simulink model "NoC_4x4x3"  (R2015a)
settings: Solver=ode45  StartTime=0.0  StopTime=10.0  RelTol=1e-3
undefined symbols (not defined in the file or in its folder): des, SELECT
undefined symbols (not defined in the file): MAX, MIN, T
libraries: simulink x48
(part 1 of 12)
settings Model: Creator=Nejib  LastModifiedBy=Nejib

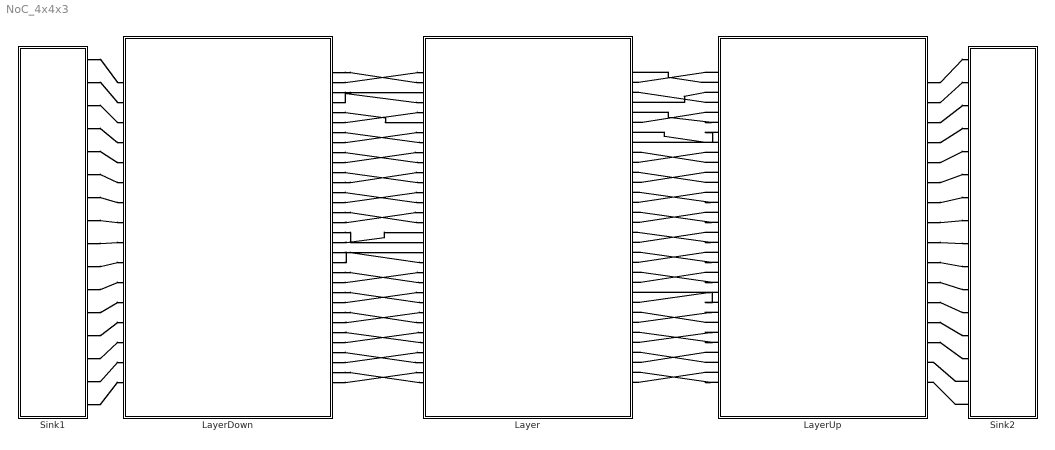
== system NoC_4x4x3 ==
  Layer : Subsystem
  LayerDown : Subsystem
  LayerUp : Subsystem
  Sink1 : Subsystem
      mask Display: fprintf('SINK')
  Sink2 : Subsystem
      mask Display: fprintf('SINK')
  connections:
  LayerUp/LConn1 -- Layer/RConn2
  LayerUp/LConn2 -- Layer/RConn1
  LayerUp/LConn3 -- Layer/RConn4
  LayerUp/LConn4 -- Layer/RConn3
  LayerUp/LConn5 -- Layer/RConn6
  LayerUp/LConn6 -- Layer/RConn5
  LayerUp/LConn7 -- Layer/RConn8
  LayerUp/LConn8 -- Layer/RConn7
  LayerUp/LConn9 -- Layer/RConn10
  LayerUp/LConn10 -- Layer/RConn9
  LayerUp/LConn11 -- Layer/RConn12
  LayerUp/LConn12 -- Layer/RConn11
  LayerUp/LConn13 -- Layer/RConn14
  LayerUp/LConn14 -- Layer/RConn13
  LayerUp/LConn16 -- Layer/RConn15
  LayerUp/LConn15 -- Layer/RConn16
  LayerUp/LConn17 -- Layer/RConn18
  LayerUp/LConn18 -- Layer/RConn17
  LayerUp/LConn19 -- Layer/RConn20
  LayerUp/LConn20 -- Layer/RConn19
  LayerUp/LConn21 -- Layer/RConn22
  LayerUp/LConn22 -- Layer/RConn21
  LayerUp/LConn24 -- Layer/RConn23
  LayerUp/LConn23 -- Layer/RConn24
  LayerUp/LConn25 -- Layer/RConn26
  LayerUp/LConn26 -- Layer/RConn25
  LayerUp/LConn27 -- Layer/RConn28
  LayerUp/LConn28 -- Layer/RConn27
  LayerUp/LConn29 -- Layer/RConn30
  LayerUp/LConn30 -- Layer/RConn29
  LayerUp/LConn31 -- Layer/RConn32
  LayerUp/LConn32 -- Layer/RConn31
  LayerDown/RConn27 -- Layer/LConn28
  LayerDown/RConn25 -- Layer/LConn26
  LayerDown/RConn18 -- Layer/LConn17
  LayerDown/RConn12 -- Layer/LConn11
  LayerDown/RConn21 -- Layer/LConn22
  LayerDown/RConn10 -- Layer/LConn9
  LayerDown/RConn14 -- Layer/LConn13
  LayerDown/RConn32 -- Layer/LConn31
  LayerDown/RConn5 -- Layer/LConn6
  LayerDown/RConn23 -- Layer/LConn24
  LayerDown/RConn19 -- Layer/LConn20
  LayerDown/RConn15 -- Layer/LConn16
  LayerDown/RConn6 -- Layer/LConn5
  LayerDown/RConn2 -- Layer/LConn1
  LayerDown/RConn1 -- Layer/LConn2
  LayerDown/RConn3 -- Layer/LConn4
  LayerDown/RConn4 -- Layer/LConn3
  LayerDown/RConn8 -- Layer/LConn7
  LayerDown/RConn7 -- Layer/LConn8
  LayerDown/RConn9 -- Layer/LConn10
  LayerDown/RConn11 -- Layer/LConn12
  LayerDown/RConn13 -- Layer/LConn14
  LayerDown/RConn16 -- Layer/LConn15
  LayerDown/RConn17 -- Layer/LConn18
  LayerDown/RConn20 -- Layer/LConn19
  LayerDown/RConn22 -- Layer/LConn21
  LayerDown/RConn24 -- Layer/LConn23
  LayerDown/RConn26 -- Layer/LConn25
  LayerDown/RConn28 -- Layer/LConn27
  LayerDown/RConn30 -- Layer/LConn29
  LayerDown/RConn29 -- Layer/LConn30
  LayerDown/RConn31 -- Layer/LConn32
  LayerUp/RConn2 -- Sink2/LConn1
  LayerUp/RConn4 -- Sink2/LConn2
  LayerUp/RConn6 -- Sink2/LConn3
  LayerUp/RConn8 -- Sink2/LConn4
  LayerUp/RConn10 -- Sink2/LConn5
  LayerUp/RConn12 -- Sink2/LConn6
  LayerUp/RConn14 -- Sink2/LConn7
  LayerUp/RConn16 -- Sink2/LConn8
  LayerUp/RConn18 -- Sink2/LConn9
  LayerUp/RConn20 -- Sink2/LConn10
  LayerUp/RConn22 -- Sink2/LConn11
  LayerUp/RConn24 -- Sink2/LConn12
  LayerUp/RConn26 -- Sink2/LConn13
  LayerUp/RConn28 -- Sink2/LConn14
  Sink2/LConn15 -- LayerUp/RConn30
  Sink2/LConn16 -- LayerUp/RConn32
  Sink1/LConn1 -- LayerDown/LConn2
  Sink1/LConn2 -- LayerDown/LConn4
  Sink1/LConn3 -- LayerDown/LConn6
  Sink1/LConn4 -- LayerDown/LConn8
  Sink1/LConn5 -- LayerDown/LConn10
  Sink1/LConn6 -- LayerDown/LConn12
  Sink1/LConn7 -- LayerDown/LConn14
  Sink1/LConn8 -- LayerDown/LConn16
  Sink1/LConn9 -- LayerDown/LConn18
  Sink1/LConn10 -- LayerDown/LConn20
  Sink1/LConn11 -- LayerDown/LConn22
  Sink1/LConn12 -- LayerDown/LConn24
  Sink1/LConn13 -- LayerDown/LConn26
  Sink1/LConn14 -- LayerDown/LConn28
  Sink1/LConn15 -- LayerDown/LConn30
  Sink1/LConn16 -- LayerDown/LConn32

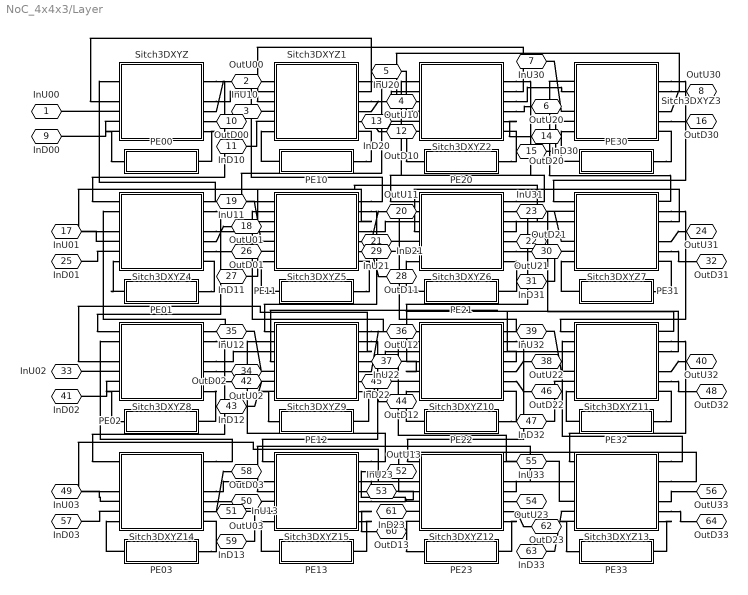
== system NoC_4x4x3/Layer ==
  PE00 : Subsystem  mask{ME=[1 1 2], D=5, SEED=100, tt=Uniform, MINU=MIN, MAXU=MAX, REGULAR=T, A=100, B=15, Router='Corner_Mean_Z2', Loss='Corner_Loss_Z2', N='Corner_N_Z2'}
      mask prompts: ME "Addresse"; D "Startup time"; tt "Traffic Type"; MINU "Min"; MAXU "Max"; REGULAR "T"; A "Lambda 1"; B "Lambda 2"; Router "Mean delay"; Loss "Instant number of lost flits"; N "Number of departed flits"
      mask init:
      | set_param([gcb '/Router'],'VariableName',Router)
      | set_param([gcb '/Loss'],'VariableName',Loss)
      | set_param([gcb '/N'],'VariableName',N)
      | V=1:4;
      | V_X = V(V~=ME(1));
      | V_Y = V(V~=ME(2));
      | V_Z = V(V~=ME(3));
      mask TypeOptions tt: Periodic | Uniform | MMPP
      mask Callback tt:
      | maskStr = get_param(gcb,'tt');
      | msk = Simulink.Mask.get(gcbh);
      | %p = msk.Parameters;
      | %
      | % P = msk.getParameter('MINU');
      | % U = msk.getParameter('MAXU');
      | % M = msk.getParameter('REGULAR');
      | 
      | P = msk.getDialogControl('Periodic');
      | U = msk.getDialogControl('Uniform');
      | M = msk.getDialogControl('MMPP');
      | 
      | % The pop-up menu is the first mask parameter.
      | %   Check the value selected in the pop-up
      | if strcmp(maskStr(1),'P'),
      | 
      |     % Set the visibility of both parameters on when
      |     %   User-defined is selected in the pop-up.
      |     %set_param(gcb,'MaskValues',{'Default','1','1'})
      |     %set_param(gcb,'MaskVisibilities','off'),
      |     SELECT = 1;
      |     P.Visible= 'on';
      |     U.Visible= 'off';
      |     M.Visible= 'off';
      | 
      | elseif strcmp(maskStr(1),'U'),
      |     P.Visible= 'off';
      |     U.Visible= 'on';
      |     M.Visible= 'off';
      | 
      |     SELECT = 2;
      | else
      |     P.Visible= 'off';
      |     U.Visible= 'off';
      |     M.Visible= 'on';
      | 
      |     SELECT = 3;
      | end
      mask DialogControl DescTextVar Prompt: Generates traffic from a given adress using one of three possible traffic patterns: Periodic, Uniform and Markov Modulated Poisson Process.
  PE01 : Subsystem  mask{ME=[1 2  2], D=5, SEED=100, tt=Uniform, MINU=MIN, MAXU=MAX, REGULAR=T, A=100, B=15, Router='Side_Mean_Z2', Loss='Side_Loss_Z2', N='Side_N_Z2'}
      mask prompts: ME "Addresse"; D "Startup time"; tt "Traffic Type"; MINU "Min"; MAXU "Max"; REGULAR "T"; A "Lambda 1"; B "Lambda 2"; Router "Mean delay"; Loss "Instant number of lost flits"; N "Number of departed flits"
      mask init:
      | %set_param([gcb '/Inst'],'VariableName',Inst)
      | set_param([gcb '/Router'],'VariableName',Router)
      | set_param([gcb '/Loss'],'VariableName',Loss)
      | set_param([gcb '/N'],'VariableName',N)
      | V=1:4;
      | V_X = V(V~=ME(1));
      | V_Y = V(V~=ME(2));
      | V_Z = V(V~=ME(3));
      mask TypeOptions tt: Periodic | Uniform | MMPP
      mask Callback tt:
      | maskStr = get_param(gcb,'tt');
      | msk = Simulink.Mask.get(gcbh);
      | %p = msk.Parameters;
      | %
      | % P = msk.getParameter('MINU');
      | % U = msk.getParameter('MAXU');
      | % M = msk.getParameter('REGULAR');
      | 
      | P = msk.getDialogControl('Periodic');
      | U = msk.getDialogControl('Uniform');
      | M = msk.getDialogControl('MMPP');
      | 
      | % The pop-up menu is the first mask parameter.
      | %   Check the value selected in the pop-up
      | if strcmp(maskStr(1),'P'),
      | 
      |     % Set the visibility of both parameters on when
      |     %   User-defined is selected in the pop-up.
      |     %set_param(gcb,'MaskValues',{'Default','1','1'})
      |     %set_param(gcb,'MaskVisibilities','off'),
      |     SELECT = 1;
      |     P.Visible= 'on';
      |     U.Visible= 'off';
      |     M.Visible= 'off';
      | 
      | elseif strcmp(maskStr(1),'U'),
      |     P.Visible= 'off';
      |     U.Visible= 'on';
      |     M.Visible= 'off';
      | 
      |     SELECT = 2;
      | else
      |     P.Visible= 'off';
      |     U.Visible= 'off';
      |     M.Visible= 'on';
      | 
      |     SELECT = 3;
      | end
      mask DialogControl DescTextVar Prompt: Generates traffic from a given adress using one of three possible traffic patterns: Periodic, Uniform and Markov Modulated Poisson Process.
  PE02 : Subsystem  mask{ME=[1 3 2], D=5, SEED=100, tt=Uniform, MINU=MIN, MAXU=MAX, REGULAR=T, A=100, B=15}
      mask prompts: ME "Addresse"; D "Startup time"; tt "Traffic Type"; MINU "Min"; MAXU "Max"; REGULAR "T"; A "Lambda 1"; B "Lambda 2"
      mask init:
      | V=1:4;
      | V_X = V(V~=ME(1));
      | V_Y = V(V~=ME(2));
      | V=1:3;
      | V_Z = V(V~=ME(3));
      mask TypeOptions tt: Periodic | Uniform | MMPP
      mask Callback tt:
      | maskStr = get_param(gcb,'tt');
      | msk = Simulink.Mask.get(gcbh);
      | %p = msk.Parameters;
      | %
      | % P = msk.getParameter('MINU');
      | % U = msk.getParameter('MAXU');
      | % M = msk.getParameter('REGULAR');
      | 
      | P = msk.getDialogControl('Periodic');
      | U = msk.getDialogControl('Uniform');
      | M = msk.getDialogControl('MMPP');
      | 
      | % The pop-up menu is the first mask parameter.
      | %   Check the value selected in the pop-up
      | if strcmp(maskStr(1),'P'),
      | 
      |     % Set the visibility of both parameters on when
      |     %   User-defined is selected in the pop-up.
      |     %set_param(gcb,'MaskValues',{'Default','1','1'})
      |     %set_param(gcb,'MaskVisibilities','off'),
      |     SELECT = 1;
      |     P.Visible= 'on';
      |     U.Visible= 'off';
      |     M.Visible= 'off';
      | 
      | elseif strcmp(maskStr(1),'U'),
      |     P.Visible= 'off';
      |     U.Visible= 'on';
      |     M.Visible= 'off';
      | 
      |     SELECT = 2;
      | else
      |     P.Visible= 'off';
      |     U.Visible= 'off';
      |     M.Visible= 'on';
      | 
      |     SELECT = 3;
      | end
      mask DialogControl DescTextVar Prompt: Generates traffic from a given adress using one of three possible traffic patterns: Periodic, Uniform and Markov Modulated Poisson Process.
  PE03 : Subsystem  mask{ME=[1 4 2], D=5, SEED=100, tt=Uniform, MINU=MIN, MAXU=MAX, REGULAR=T, A=100, B=15}
      mask prompts: ME "Addresse"; D "Startup time"; tt "Traffic Type"; MINU "Min"; MAXU "Max"; REGULAR "T"; A "Lambda 1"; B "Lambda 2"
      mask init:
      | V=1:4;
      | V_X = V(V~=ME(1));
      | V_Y = V(V~=ME(2));
      | V=1:3;
      | V_Z = V(V~=ME(3));
      mask TypeOptions tt: Periodic | Uniform | MMPP
      mask Callback tt:
      | maskStr = get_param(gcb,'tt');
      | msk = Simulink.Mask.get(gcbh);
      | %p = msk.Parameters;
      | %
      | % P = msk.getParameter('MINU');
      | % U = msk.getParameter('MAXU');
      | % M = msk.getParameter('REGULAR');
      | 
      | P = msk.getDialogControl('Periodic');
      | U = msk.getDialogControl('Uniform');
      | M = msk.getDialogControl('MMPP');
      | 
      | % The pop-up menu is the first mask parameter.
      | %   Check the value selected in the pop-up
      | if strcmp(maskStr(1),'P'),
      | 
      |     % Set the visibility of both parameters on when
      |     %   User-defined is selected in the pop-up.
      |     %set_param(gcb,'MaskValues',{'Default','1','1'})
      |     %set_param(gcb,'MaskVisibilities','off'),
      |     SELECT = 1;
      |     P.Visible= 'on';
      |     U.Visible= 'off';
      |     M.Visible= 'off';
      | 
      | elseif strcmp(maskStr(1),'U'),
      |     P.Visible= 'off';
      |     U.Visible= 'on';
      |     M.Visible= 'off';
      | 
      |     SELECT = 2;
      | else
      |     P.Visible= 'off';
      |     U.Visible= 'off';
      |     M.Visible= 'on';
      | 
      |     SELECT = 3;
      | end
      mask DialogControl DescTextVar Prompt: Generates traffic from a given adress using one of three possible traffic patterns: Periodic, Uniform and Markov Modulated Poisson Process.
  PE10 : Subsystem  mask{ME=[2 1 2], D=5, SEED=100, tt=Uniform, MINU=MIN, MAXU=MAX, REGULAR=1, A=100, B=15}
      mask prompts: ME "Addresse"; D "Startup time"; tt "Traffic Type"; MINU "Min"; MAXU "Max"; REGULAR "T"; A "Lambda 1"; B "Lambda 2"
      mask init:
      | V=1:4;
      | V_X = V(V~=ME(1));
      | V_Y = V(V~=ME(2));
      | V=1:3;
      | V_Z = V(V~=ME(3));
      mask TypeOptions tt: Periodic | Uniform | MMPP
      mask Callback tt:
      | maskStr = get_param(gcb,'tt');
      | msk = Simulink.Mask.get(gcbh);
      | %p = msk.Parameters;
      | %
      | % P = msk.getParameter('MINU');
      | % U = msk.getParameter('MAXU');
      | % M = msk.getParameter('REGULAR');
      | 
      | P = msk.getDialogControl('Periodic');
      | U = msk.getDialogControl('Uniform');
      | M = msk.getDialogControl('MMPP');
      | 
      | % The pop-up menu is the first mask parameter.
      | %   Check the value selected in the pop-up
      | if strcmp(maskStr(1),'P'),
      | 
      |     % Set the visibility of both parameters on when
      |     %   User-defined is selected in the pop-up.
      |     %set_param(gcb,'MaskValues',{'Default','1','1'})
      |     %set_param(gcb,'MaskVisibilities','off'),
      |     SELECT = 1;
      |     P.Visible= 'on';
      |     U.Visible= 'off';
      |     M.Visible= 'off';
      | 
      | elseif strcmp(maskStr(1),'U'),
      |     P.Visible= 'off';
      |     U.Visible= 'on';
      |     M.Visible= 'off';
      | 
      |     SELECT = 2;
      | else
      |     P.Visible= 'off';
      |     U.Visible= 'off';
      |     M.Visible= 'on';
      | 
      |     SELECT = 3;
      | end
      mask DialogControl DescTextVar Prompt: Generates traffic from a given adress using one of three possible traffic patterns: Periodic, Uniform and Markov Modulated Poisson Process.
  PE11 : Subsystem  mask{ME=[2 2 2], D=5, SEED=100, tt=Uniform, MINU=MIN, MAXU=MAX, REGULAR=T, A=100, B=15, Router='Midlle_Mean_Z2', Loss='Midlle_Loss_Z2', N='Midlle_N_Z2'}
      mask prompts: ME "Addresse"; D "Startup time"; tt "Traffic Type"; MINU "Min"; MAXU "Max"; REGULAR "T"; A "Lambda 1"; B "Lambda 2"; Router "Mean delay"; Loss "Instant number of lost flits"; N "Number of departed flits"
      mask init:
      | %et_param([gcb '/Inst'],'VariableName',Inst)
      | set_param([gcb '/Router'],'VariableName',Router)
      | set_param([gcb '/Loss'],'VariableName',Loss)
      | set_param([gcb '/N'],'VariableName',N)
      | V=1:4;
      | V_X = V(V~=ME(1));
      | V_Y = V(V~=ME(2));
      | V_Z = V(V~=ME(3));
      mask TypeOptions tt: Periodic | Uniform | MMPP
      mask Callback tt:
      | maskStr = get_param(gcb,'tt');
      | msk = Simulink.Mask.get(gcbh);
      | %p = msk.Parameters;
      | %
      | % P = msk.getParameter('MINU');
      | % U = msk.getParameter('MAXU');
      | % M = msk.getParameter('REGULAR');
      | 
      | P = msk.getDialogControl('Periodic');
      | U = msk.getDialogControl('Uniform');
      | M = msk.getDialogControl('MMPP');
      | 
      | % The pop-up menu is the first mask parameter.
      | %   Check the value selected in the pop-up
      | if strcmp(maskStr(1),'P'),
      | 
      |     % Set the visibility of both parameters on when
      |     %   User-defined is selected in the pop-up.
      |     %set_param(gcb,'MaskValues',{'Default','1','1'})
      |     %set_param(gcb,'MaskVisibilities','off'),
      |     SELECT = 1;
      |     P.Visible= 'on';
      |     U.Visible= 'off';
      |     M.Visible= 'off';
      | 
      | elseif strcmp(maskStr(1),'U'),
      |     P.Visible= 'off';
      |     U.Visible= 'on';
      |     M.Visible= 'off';
      | 
      |     SELECT = 2;
      | else
      |     P.Visible= 'off';
      |     U.Visible= 'off';
      |     M.Visible= 'on';
      | 
      |     SELECT = 3;
      | end
      mask DialogControl DescTextVar Prompt: Generates traffic from a given adress using one of three possible traffic patterns: Periodic, Uniform and Markov Modulated Poisson Process.
  PE12 : Subsystem  mask{ME=[2 3 2], D=5, SEED=100, tt=Uniform, MINU=MIN, MAXU=MAX, REGULAR=T, A=100, B=15}
      mask prompts: ME "Addresse"; D "Startup time"; tt "Traffic Type"; MINU "Min"; MAXU "Max"; REGULAR "T"; A "Lambda 1"; B "Lambda 2"
      mask init:
      | V=1:4;
      | V_X = V(V~=ME(1));
      | V_Y = V(V~=ME(2));
      | V=1:3;
      | V_Z = V(V~=ME(3));
      mask TypeOptions tt: Periodic | Uniform | MMPP
      mask Callback tt:
      | maskStr = get_param(gcb,'tt');
      | msk = Simulink.Mask.get(gcbh);
      | %p = msk.Parameters;
      | %
      | % P = msk.getParameter('MINU');
      | % U = msk.getParameter('MAXU');
      | % M = msk.getParameter('REGULAR');
      | 
      | P = msk.getDialogControl('Periodic');
      | U = msk.getDialogControl('Uniform');
      | M = msk.getDialogControl('MMPP');
      | 
      | % The pop-up menu is the first mask parameter.
      | %   Check the value selected in the pop-up
      | if strcmp(maskStr(1),'P'),
      | 
      |     % Set the visibility of both parameters on when
      |     %   User-defined is selected in the pop-up.
      |     %set_param(gcb,'MaskValues',{'Default','1','1'})
      |     %set_param(gcb,'MaskVisibilities','off'),
      |     SELECT = 1;
      |     P.Visible= 'on';
      |     U.Visible= 'off';
      |     M.Visible= 'off';
      | 
      | elseif strcmp(maskStr(1),'U'),
      |     P.Visible= 'off';
      |     U.Visible= 'on';
      |     M.Visible= 'off';
      | 
      |     SELECT = 2;
      | else
      |     P.Visible= 'off';
      |     U.Visible= 'off';
      |     M.Visible= 'on';
      | 
      |     SELECT = 3;
      | end
      mask DialogControl DescTextVar Prompt: Generates traffic from a given adress using one of three possible traffic patterns: Periodic, Uniform and Markov Modulated Poisson Process.
  PE13 : Subsystem  mask{ME=[2 4 2], D=5, SEED=100, tt=Uniform, MINU=MIN, MAXU=MAX, REGULAR=T, A=100, B=15}
      mask prompts: ME "Addresse"; D "Startup time"; tt "Traffic Type"; MINU "Min"; MAXU "Max"; REGULAR "T"; A "Lambda 1"; B "Lambda 2"
      mask init:
      | V=1:4;
      | V_X = V(V~=ME(1));
      | V_Y = V(V~=ME(2));
      | V=1:3;
      | V_Z = V(V~=ME(3));
      mask TypeOptions tt: Periodic | Uniform | MMPP
      mask Callback tt:
      | maskStr = get_param(gcb,'tt');
      | msk = Simulink.Mask.get(gcbh);
      | %p = msk.Parameters;
      | %
      | % P = msk.getParameter('MINU');
      | % U = msk.getParameter('MAXU');
      | % M = msk.getParameter('REGULAR');
      | 
      | P = msk.getDialogControl('Periodic');
      | U = msk.getDialogControl('Uniform');
      | M = msk.getDialogControl('MMPP');
      | 
      | % The pop-up menu is the first mask parameter.
      | %   Check the value selected in the pop-up
      | if strcmp(maskStr(1),'P'),
      | 
      |     % Set the visibility of both parameters on when
      |     %   User-defined is selected in the pop-up.
      |     %set_param(gcb,'MaskValues',{'Default','1','1'})
      |     %set_param(gcb,'MaskVisibilities','off'),
      |     SELECT = 1;
      |     P.Visible= 'on';
      |     U.Visible= 'off';
      |     M.Visible= 'off';
      | 
      | elseif strcmp(maskStr(1),'U'),
      |     P.Visible= 'off';
      |     U.Visible= 'on';
      |     M.Visible= 'off';
      | 
      |     SELECT = 2;
      | else
      |     P.Visible= 'off';
      |     U.Visible= 'off';
      |     M.Visible= 'on';
      | 
      |     SELECT = 3;
      | end
      mask DialogControl DescTextVar Prompt: Generates traffic from a given adress using one of three possible traffic patterns: Periodic, Uniform and Markov Modulated Poisson Process.
  PE20 : Subsystem  mask{ME=[3 1 2], D=5, SEED=100, tt=Uniform, MINU=MIN, MAXU=MAX, REGULAR=T, A=100, B=15}
      mask prompts: ME "Addresse"; D "Startup time"; tt "Traffic Type"; MINU "Min"; MAXU "Max"; REGULAR "T"; A "Lambda 1"; B "Lambda 2"
      mask init:
      | V=1:4;
      | V_X = V(V~=ME(1));
      | V_Y = V(V~=ME(2));
      | V=1:3;
      | V_Z = V(V~=ME(3));
      mask TypeOptions tt: Periodic | Uniform | MMPP
      mask Callback tt:
      | maskStr = get_param(gcb,'tt');
      | msk = Simulink.Mask.get(gcbh);
      | %p = msk.Parameters;
      | %
      | % P = msk.getParameter('MINU');
      | % U = msk.getParameter('MAXU');
      | % M = msk.getParameter('REGULAR');
      | 
      | P = msk.getDialogControl('Periodic');
      | U = msk.getDialogControl('Uniform');
      | M = msk.getDialogControl('MMPP');
      | 
      | % The pop-up menu is the first mask parameter.
      | %   Check the value selected in the pop-up
      | if strcmp(maskStr(1),'P'),
      | 
      |     % Set the visibility of both parameters on when
      |     %   User-defined is selected in the pop-up.
      |     %set_param(gcb,'MaskValues',{'Default','1','1'})
      |     %set_param(gcb,'MaskVisibilities','off'),
      |     SELECT = 1;
      |     P.Visible= 'on';
      |     U.Visible= 'off';
      |     M.Visible= 'off';
      | 
      | elseif strcmp(maskStr(1),'U'),
      |     P.Visible= 'off';
      |     U.Visible= 'on';
      |     M.Visible= 'off';
      | 
      |     SELECT = 2;
      | else
      |     P.Visible= 'off';
      |     U.Visible= 'off';
      |     M.Visible= 'on';
      | 
      |     SELECT = 3;
      | end
      mask DialogControl DescTextVar Prompt: Generates traffic from a given adress using one of three possible traffic patterns: Periodic, Uniform and Markov Modulated Poisson Process.
  PE21 : Subsystem  mask{ME=[3 2 2], D=5, SEED=100, tt=Uniform, MINU=MIN, MAXU=MAX, REGULAR=T, A=100, B=15}
      mask prompts: ME "Addresse"; D "Startup time"; tt "Traffic Type"; MINU "Min"; MAXU "Max"; REGULAR "T"; A "Lambda 1"; B "Lambda 2"
      mask init:
      | V=1:4;
      | V_X = V(V~=ME(1));
      | V_Y = V(V~=ME(2));
      | V=1:3;
      | V_Z = V(V~=ME(3));
      mask TypeOptions tt: Periodic | Uniform | MMPP
      mask Callback tt:
      | maskStr = get_param(gcb,'tt');
      | msk = Simulink.Mask.get(gcbh);
      | %p = msk.Parameters;
      | %
      | % P = msk.getParameter('MINU');
      | % U = msk.getParameter('MAXU');
      | % M = msk.getParameter('REGULAR');
      | 
      | P = msk.getDialogControl('Periodic');
      | U = msk.getDialogControl('Uniform');
      | M = msk.getDialogControl('MMPP');
      | 
      | % The pop-up menu is the first mask parameter.
      | %   Check the value selected in the pop-up
      | if strcmp(maskStr(1),'P'),
      | 
      |     % Set the visibility of both parameters on when
      |     %   User-defined is selected in the pop-up.
      |     %set_param(gcb,'MaskValues',{'Default','1','1'})
      |     %set_param(gcb,'MaskVisibilities','off'),
      |     SELECT = 1;
      |     P.Visible= 'on';
      |     U.Visible= 'off';
      |     M.Visible= 'off';
      | 
      | elseif strcmp(maskStr(1),'U'),
      |     P.Visible= 'off';
      |     U.Visible= 'on';
      |     M.Visible= 'off';
      | 
      |     SELECT = 2;
      | else
      |     P.Visible= 'off';
      |     U.Visible= 'off';
      |     M.Visible= 'on';
      | 
      |     SELECT = 3;
      | end
      mask DialogControl DescTextVar Prompt: Generates traffic from a given adress using one of three possible traffic patterns: Periodic, Uniform and Markov Modulated Poisson Process.
  PE22 : Subsystem  mask{ME=[3 3 2], D=5, SEED=100, tt=Uniform, MINU=MIN, MAXU=MAX, REGULAR=T, A=100, B=15}
      mask prompts: ME "Addresse"; D "Startup time"; tt "Traffic Type"; MINU "Min"; MAXU "Max"; REGULAR "T"; A "Lambda 1"; B "Lambda 2"
      mask init:
      | V=1:4;
      | V_X = V(V~=ME(1));
      | V_Y = V(V~=ME(2));
      | V=1:3;
      | V_Z = V(V~=ME(3));
      mask TypeOptions tt: Periodic | Uniform | MMPP
      mask Callback tt:
      | maskStr = get_param(gcb,'tt');
      | msk = Simulink.Mask.get(gcbh);
      | %p = msk.Parameters;
      | %
      | % P = msk.getParameter('MINU');
      | % U = msk.getParameter('MAXU');
      | % M = msk.getParameter('REGULAR');
      | 
      | P = msk.getDialogControl('Periodic');
      | U = msk.getDialogControl('Uniform');
      | M = msk.getDialogControl('MMPP');
      | 
      | % The pop-up menu is the first mask parameter.
      | %   Check the value selected in the pop-up
      | if strcmp(maskStr(1),'P'),
      | 
      |     % Set the visibility of both parameters on when
      |     %   User-defined is selected in the pop-up.
      |     %set_param(gcb,'MaskValues',{'Default','1','1'})
      |     %set_param(gcb,'MaskVisibilities','off'),
      |     SELECT = 1;
      |     P.Visible= 'on';
      |     U.Visible= 'off';
      |     M.Visible= 'off';
      | 
      | elseif strcmp(maskStr(1),'U'),
      |     P.Visible= 'off';
      |     U.Visible= 'on';
      |     M.Visible= 'off';
      | 
      |     SELECT = 2;
      | else
      |     P.Visible= 'off';
      |     U.Visible= 'off';
      |     M.Visible= 'on';
      | 
      |     SELECT = 3;
      | end
      mask DialogControl DescTextVar Prompt: Generates traffic from a given adress using one of three possible traffic patterns: Periodic, Uniform and Markov Modulated Poisson Process.
  PE23 : Subsystem  mask{ME=[3 4 2], D=5, SEED=100, tt=Uniform, MINU=MIN, MAXU=MAX, REGULAR=T, A=100, B=15}
      mask prompts: ME "Addresse"; D "Startup time"; tt "Traffic Type"; MINU "Min"; MAXU "Max"; REGULAR "T"; A "Lambda 1"; B "Lambda 2"
      mask init:
      | V=1:4;
      | V_X = V(V~=ME(1));
      | V_Y = V(V~=ME(2));
      | V=1:3;
      | V_Z = V(V~=ME(3));
      mask TypeOptions tt: Periodic | Uniform | MMPP
      mask Callback tt:
      | maskStr = get_param(gcb,'tt');
      | msk = Simulink.Mask.get(gcbh);
      | %p = msk.Parameters;
      | %
      | % P = msk.getParameter('MINU');
      | % U = msk.getParameter('MAXU');
      | % M = msk.getParameter('REGULAR');
      | 
      | P = msk.getDialogControl('Periodic');
      | U = msk.getDialogControl('Uniform');
      | M = msk.getDialogControl('MMPP');
      | 
      | % The pop-up menu is the first mask parameter.
      | %   Check the value selected in the pop-up
      | if strcmp(maskStr(1),'P'),
      | 
      |     % Set the visibility of both parameters on when
      |     %   User-defined is selected in the pop-up.
      |     %set_param(gcb,'MaskValues',{'Default','1','1'})
      |     %set_param(gcb,'MaskVisibilities','off'),
      |     SELECT = 1;
      |     P.Visible= 'on';
      |     U.Visible= 'off';
      |     M.Visible= 'off';
      | 
      | elseif strcmp(maskStr(1),'U'),
      |     P.Visible= 'off';
      |     U.Visible= 'on';
      |     M.Visible= 'off';
      | 
      |     SELECT = 2;
      | else
      |     P.Visible= 'off';
      |     U.Visible= 'off';
      |     M.Visible= 'on';
      | 
      |     SELECT = 3;
      | end
      mask DialogControl DescTextVar Prompt: Generates traffic from a given adress using one of three possible traffic patterns: Periodic, Uniform and Markov Modulated Poisson Process.
  PE30 : Subsystem  mask{ME=[4 1 2], D=5, SEED=100, tt=Uniform, MINU=MIN, MAXU=MAX, REGULAR=T, A=100, B=15}
      mask prompts: ME "Addresse"; D "Startup time"; tt "Traffic Type"; MINU "Min"; MAXU "Max"; REGULAR "T"; A "Lambda 1"; B "Lambda 2"
      mask init:
      | V=1:4;
      | V_X = V(V~=ME(1));
      | V_Y = V(V~=ME(2));
      | V=1:3;
      | V_Z = V(V~=ME(3));
      mask TypeOptions tt: Periodic | Uniform | MMPP
      mask Callback tt:
      | maskStr = get_param(gcb,'tt');
      | msk = Simulink.Mask.get(gcbh);
      | %p = msk.Parameters;
      | %
      | % P = msk.getParameter('MINU');
      | % U = msk.getParameter('MAXU');
      | % M = msk.getParameter('REGULAR');
      | 
      | P = msk.getDialogControl('Periodic');
      | U = msk.getDialogControl('Uniform');
      | M = msk.getDialogControl('MMPP');
      | 
      | % The pop-up menu is the first mask parameter.
      | %   Check the value selected in the pop-up
      | if strcmp(maskStr(1),'P'),
      | 
      |     % Set the visibility of both parameters on when
      |     %   User-defined is selected in the pop-up.
      |     %set_param(gcb,'MaskValues',{'Default','1','1'})
      |     %set_param(gcb,'MaskVisibilities','off'),
      |     SELECT = 1;
      |     P.Visible= 'on';
      |     U.Visible= 'off';
      |     M.Visible= 'off';
      | 
      | elseif strcmp(maskStr(1),'U'),
      |     P.Visible= 'off';
      |     U.Visible= 'on';
      |     M.Visible= 'off';
      | 
      |     SELECT = 2;
      | else
      |     P.Visible= 'off';
      |     U.Visible= 'off';
      |     M.Visible= 'on';
      | 
      |     SELECT = 3;
      | end
      mask DialogControl DescTextVar Prompt: Generates traffic from a given adress using one of three possible traffic patterns: Periodic, Uniform and Markov Modulated Poisson Process.
  PE31 : Subsystem  mask{ME=[4 2 2], D=5, SEED=100, tt=Uniform, MINU=MIN, MAXU=MAX, REGULAR=T, A=100, B=15}
      mask prompts: ME "Addresse"; D "Startup time"; tt "Traffic Type"; MINU "Min"; MAXU "Max"; REGULAR "T"; A "Lambda 1"; B "Lambda 2"
      mask init:
      | V=1:4;
      | V_X = V(V~=ME(1));
      | V_Y = V(V~=ME(2));
      | V=1:3;
      | V_Z = V(V~=ME(3));
      mask TypeOptions tt: Periodic | Uniform | MMPP
      mask Callback tt:
      | maskStr = get_param(gcb,'tt');
      | msk = Simulink.Mask.get(gcbh);
      | %p = msk.Parameters;
      | %
      | % P = msk.getParameter('MINU');
      | % U = msk.getParameter('MAXU');
      | % M = msk.getParameter('REGULAR');
      | 
      | P = msk.getDialogControl('Periodic');
      | U = msk.getDialogControl('Uniform');
      | M = msk.getDialogControl('MMPP');
      | 
      | % The pop-up menu is the first mask parameter.
      | %   Check the value selected in the pop-up
      | if strcmp(maskStr(1),'P'),
      | 
      |     % Set the visibility of both parameters on when
      |     %   User-defined is selected in the pop-up.
      |     %set_param(gcb,'MaskValues',{'Default','1','1'})
      |     %set_param(gcb,'MaskVisibilities','off'),
      |     SELECT = 1;
      |     P.Visible= 'on';
      |     U.Visible= 'off';
      |     M.Visible= 'off';
      | 
      | elseif strcmp(maskStr(1),'U'),
      |     P.Visible= 'off';
      |     U.Visible= 'on';
      |     M.Visible= 'off';
      | 
      |     SELECT = 2;
      | else
      |     P.Visible= 'off';
      |     U.Visible= 'off';
      |     M.Visible= 'on';
      | 
      |     SELECT = 3;
      | end
      mask DialogControl DescTextVar Prompt: Generates traffic from a given adress using one of three possible traffic patterns: Periodic, Uniform and Markov Modulated Poisson Process.
  PE32 : Subsystem  mask{ME=[4 3 2], D=5, SEED=100, tt=Uniform, MINU=MIN, MAXU=MAX, REGULAR=T, A=100, B=15}
      mask prompts: ME "Addresse"; D "Startup time"; tt "Traffic Type"; MINU "Min"; MAXU "Max"; REGULAR "T"; A "Lambda 1"; B "Lambda 2"
      mask init:
      | V=1:4;
      | V_X = V(V~=ME(1));
      | V_Y = V(V~=ME(2));
      | V=1:3;
      | V_Z = V(V~=ME(3));
      mask TypeOptions tt: Periodic | Uniform | MMPP
      mask Callback tt:
      | maskStr = get_param(gcb,'tt');
      | msk = Simulink.Mask.get(gcbh);
      | %p = msk.Parameters;
      | %
      | % P = msk.getParameter('MINU');
      | % U = msk.getParameter('MAXU');
      | % M = msk.getParameter('REGULAR');
      | 
      | P = msk.getDialogControl('Periodic');
      | U = msk.getDialogControl('Uniform');
      | M = msk.getDialogControl('MMPP');
      | 
      | % The pop-up menu is the first mask parameter.
      | %   Check the value selected in the pop-up
      | if strcmp(maskStr(1),'P'),
      | 
      |     % Set the visibility of both parameters on when
      |     %   User-defined is selected in the pop-up.
      |     %set_param(gcb,'MaskValues',{'Default','1','1'})
      |     %set_param(gcb,'MaskVisibilities','off'),
      |     SELECT = 1;
      |     P.Visible= 'on';
      |     U.Visible= 'off';
      |     M.Visible= 'off';
      | 
      | elseif strcmp(maskStr(1),'U'),
      |     P.Visible= 'off';
      |     U.Visible= 'on';
      |     M.Visible= 'off';
      | 
      |     SELECT = 2;
      | else
      |     P.Visible= 'off';
      |     U.Visible= 'off';
      |     M.Visible= 'on';
      | 
      |     SELECT = 3;
      | end
      mask DialogControl DescTextVar Prompt: Generates traffic from a given adress using one of three possible traffic patterns: Periodic, Uniform and Markov Modulated Poisson Process.
  PE33 : Subsystem  mask{ME=[4 4 2], D=5, SEED=100, tt=Uniform, MINU=MIN, MAXU=MAX, REGULAR=T, A=100, B=15}
      mask prompts: ME "Addresse"; D "Startup time"; tt "Traffic Type"; MINU "Min"; MAXU "Max"; REGULAR "T"; A "Lambda 1"; B "Lambda 2"
      mask init:
      | V=1:4;
      | V_X = V(V~=ME(1));
      | V_Y = V(V~=ME(2));
      | V=1:3;
      | V_Z = V(V~=ME(3));
      mask TypeOptions tt: Periodic | Uniform | MMPP
      mask Callback tt:
      | maskStr = get_param(gcb,'tt');
      | msk = Simulink.Mask.get(gcbh);
      | %p = msk.Parameters;
      | %
      | % P = msk.getParameter('MINU');
      | % U = msk.getParameter('MAXU');
      | % M = msk.getParameter('REGULAR');
      | 
      | P = msk.getDialogControl('Periodic');
      | U = msk.getDialogControl('Uniform');
      | M = msk.getDialogControl('MMPP');
      | 
      | % The pop-up menu is the first mask parameter.
      | %   Check the value selected in the pop-up
      | if strcmp(maskStr(1),'P'),
      | 
      |     % Set the visibility of both parameters on when
      |     %   User-defined is selected in the pop-up.
      |     %set_param(gcb,'MaskValues',{'Default','1','1'})
      |     %set_param(gcb,'MaskVisibilities','off'),
      |     SELECT = 1;
      |     P.Visible= 'on';
      |     U.Visible= 'off';
      |     M.Visible= 'off';
      | 
      | elseif strcmp(maskStr(1),'U'),
      |     P.Visible= 'off';
      |     U.Visible= 'on';
      |     M.Visible= 'off';
      | 
      |     SELECT = 2;
      | else
      |     P.Visible= 'off';
      |     U.Visible= 'off';
      |     M.Visible= 'on';
      | 
      |     SELECT = 3;
      | end
      mask DialogControl DescTextVar Prompt: Generates traffic from a given adress using one of three possible traffic patterns: Periodic, Uniform and Markov Modulated Poisson Process.
  Sitch3DXYZ : Subsystem  mask{ME_X=1, ME_Y=1, ME_Z=2, C=16, D=1, F=1, S=1e-6}
      mask prompts: ME_X "X"; ME_Y "Y"; ME_Z "Z"; C "Input FIFO size in flits"; D "Routing and arbitration delay"; F "Clock Frequency"; S "Standard Deviation"
      mask DialogControl DescTextVar Prompt: 7 Port router with the XYZ routing algorithm.
      mask DialogControl Container6 Prompt: Address
  Sitch3DXYZ1 : Subsystem  mask{ME_X=2, ME_Y=1, ME_Z=2, C=16, D=1, F=1, S=1e-6}
      mask prompts: ME_X "X"; ME_Y "Y"; ME_Z "Z"; C "Input FIFO size in flits"; D "Routing and arbitration delay"; F "Clock Frequency"; S "Standard Deviation"
      mask DialogControl DescTextVar Prompt: 7 Port router with the XYZ routing algorithm.
      mask DialogControl Container6 Prompt: Address
  Sitch3DXYZ10 : Subsystem  mask{ME_X=3, ME_Y=3, ME_Z=2, C=16, D=1, F=1, S=1e-6}
      mask prompts: ME_X "X"; ME_Y "Y"; ME_Z "Z"; C "Input FIFO size in flits"; D "Routing and arbitration delay"; F "Clock Frequency"; S "Standard Deviation"
      mask DialogControl DescTextVar Prompt: 7 Port router with the XYZ routing algorithm.
      mask DialogControl Container6 Prompt: Address
  Sitch3DXYZ11 : Subsystem  mask{ME_X=4, ME_Y=3, ME_Z=2, C=16, D=1, F=1, S=1e-6}
      mask prompts: ME_X "X"; ME_Y "Y"; ME_Z "Z"; C "Input FIFO size in flits"; D "Routing and arbitration delay"; F "Clock Frequency"; S "Standard Deviation"
      mask DialogControl DescTextVar Prompt: 7 Port router with the XYZ routing algorithm.
      mask DialogControl Container6 Prompt: Address
  Sitch3DXYZ12 : Subsystem  mask{ME_X=3, ME_Y=4, ME_Z=2, C=16, D=1, F=1, S=1e-6}
      mask prompts: ME_X "X"; ME_Y "Y"; ME_Z "Z"; C "Input FIFO size in flits"; D "Routing and arbitration delay"; F "Clock Frequency"; S "Standard Deviation"
      mask DialogControl DescTextVar Prompt: 7 Port router with the XYZ routing algorithm.
      mask DialogControl Container6 Prompt: Address
  Sitch3DXYZ13 : Subsystem  mask{ME_X=4, ME_Y=4, ME_Z=2, C=16, D=1, F=1, S=1e-6}
      mask prompts: ME_X "X"; ME_Y "Y"; ME_Z "Z"; C "Input FIFO size in flits"; D "Routing and arbitration delay"; F "Clock Frequency"; S "Standard Deviation"
      mask DialogControl DescTextVar Prompt: 7 Port router with the XYZ routing algorithm.
      mask DialogControl Container6 Prompt: Address
  Sitch3DXYZ14 : Subsystem  mask{ME_X=1, ME_Y=4, ME_Z=2, C=16, D=1, F=1, S=1e-6}
      mask prompts: ME_X "X"; ME_Y "Y"; ME_Z "Z"; C "Input FIFO size in flits"; D "Routing and arbitration delay"; F "Clock Frequency"; S "Standard Deviation"
      mask DialogControl DescTextVar Prompt: 7 Port router with the XYZ routing algorithm.
      mask DialogControl Container6 Prompt: Address
  Sitch3DXYZ15 : Subsystem  mask{ME_X=2, ME_Y=4, ME_Z=2, C=16, D=1, F=1, S=1e-6}
      mask prompts: ME_X "X"; ME_Y "Y"; ME_Z "Z"; C "Input FIFO size in flits"; D "Routing and arbitration delay"; F "Clock Frequency"; S "Standard Deviation"
      mask DialogControl DescTextVar Prompt: 7 Port router with the XYZ routing algorithm.
      mask DialogControl Container6 Prompt: Address
  Sitch3DXYZ2 : Subsystem  mask{ME_X=3, ME_Y=1, ME_Z=2, C=16, D=1, F=1, S=1e-6}
      mask prompts: ME_X "X"; ME_Y "Y"; ME_Z "Z"; C "Input FIFO size in flits"; D "Routing and arbitration delay"; F "Clock Frequency"; S "Standard Deviation"
      mask DialogControl DescTextVar Prompt: 7 Port router with the XYZ routing algorithm.
      mask DialogControl Container6 Prompt: Address
  Sitch3DXYZ3 : Subsystem  mask{ME_X=4, ME_Y=1, ME_Z=2, C=16, D=1, F=1, S=1e-6}
      mask prompts: ME_X "X"; ME_Y "Y"; ME_Z "Z"; C "Input FIFO size in flits"; D "Routing and arbitration delay"; F "Clock Frequency"; S "Standard Deviation"
      mask DialogControl DescTextVar Prompt: 7 Port router with the XYZ routing algorithm.
      mask DialogControl Container6 Prompt: Address
  Sitch3DXYZ4 : Subsystem  mask{ME_X=1, ME_Y=2, ME_Z=2, C=16, D=1, F=1, S=1e-6}
      mask prompts: ME_X "X"; ME_Y "Y"; ME_Z "Z"; C "Input FIFO size in flits"; D "Routing and arbitration delay"; F "Clock Frequency"; S "Standard Deviation"
      mask DialogControl DescTextVar Prompt: 7 Port router with the XYZ routing algorithm.
      mask DialogControl Container6 Prompt: Address
  Sitch3DXYZ5 : Subsystem  mask{ME_X=2, ME_Y=2, ME_Z=2, C=16, D=1, F=1, S=1e-6}
      mask prompts: ME_X "X"; ME_Y "Y"; ME_Z "Z"; C "Input FIFO size in flits"; D "Routing and arbitration delay"; F "Clock Frequency"; S "Standard Deviation"
      mask DialogControl DescTextVar Prompt: 7 Port router with the XYZ routing algorithm.
      mask DialogControl Container6 Prompt: Address
  Sitch3DXYZ6 : Subsystem  mask{ME_X=3, ME_Y=2, ME_Z=2, C=16, D=1, F=1, S=1e-6}
      mask prompts: ME_X "X"; ME_Y "Y"; ME_Z "Z"; C "Input FIFO size in flits"; D "Routing and arbitration delay"; F "Clock Frequency"; S "Standard Deviation"
      mask DialogControl DescTextVar Prompt: 7 Port router with the XYZ routing algorithm.
      mask DialogControl Container6 Prompt: Address
  Sitch3DXYZ7 : Subsystem  mask{ME_X=4, ME_Y=2, ME_Z=2, C=16, D=1, F=1, S=1e-6}
      mask prompts: ME_X "X"; ME_Y "Y"; ME_Z "Z"; C "Input FIFO size in flits"; D "Routing and arbitration delay"; F "Clock Frequency"; S "Standard Deviation"
      mask DialogControl DescTextVar Prompt: 7 Port router with the XYZ routing algorithm.
      mask DialogControl Container6 Prompt: Address
  Sitch3DXYZ8 : Subsystem  mask{ME_X=1, ME_Y=3, ME_Z=2, C=16, D=1, F=1, S=1e-6}
      mask prompts: ME_X "X"; ME_Y "Y"; ME_Z "Z"; C "Input FIFO size in flits"; D "Routing and arbitration delay"; F "Clock Frequency"; S "Standard Deviation"
      mask DialogControl DescTextVar Prompt: 7 Port router with the XYZ routing algorithm.
      mask DialogControl Container6 Prompt: Address
  Sitch3DXYZ9 : Subsystem  mask{ME_X=2, ME_Y=3, ME_Z=2, C=16, D=1, F=1, S=1e-6}
      mask prompts: ME_X "X"; ME_Y "Y"; ME_Z "Z"; C "Input FIFO size in flits"; D "Routing and arbitration delay"; F "Clock Frequency"; S "Standard Deviation"
      mask DialogControl DescTextVar Prompt: 7 Port router with the XYZ routing algorithm.
      mask DialogControl Container6 Prompt: Address
  InU00 : PMIOPort  Port=1  Side=Right
  OutU00 : PMIOPort  Port=2  Side=Right
  InU10 : PMIOPort  Port=3  Side=Right
  OutU10 : PMIOPort  Port=4  Side=Right
  InU20 : PMIOPort  Port=5  Side=Right
  OutU20 : PMIOPort  Port=6  Side=Right
  InU30 : PMIOPort  Port=7  Side=Right
  OutU30 : PMIOPort  Port=8  Side=Right
  InD00 : PMIOPort  Port=9  Side=Left
  OutD00 : PMIOPort  Port=10  Side=Left
  InD10 : PMIOPort  Port=11  Side=Left
  OutD10 : PMIOPort  Port=12  Side=Left
  InD20 : PMIOPort  Port=13  Side=Left
  OutD20 : PMIOPort  Port=14  Side=Left
  InD30 : PMIOPort  Port=15  Side=Left
  OutD30 : PMIOPort  Port=16  Side=Left
  InU01 : PMIOPort  Port=17  Side=Right
  OutU01 : PMIOPort  Port=18  Side=Right
  InU11 : PMIOPort  Port=19  Side=Right
  OutU11 : PMIOPort  Port=20  Side=Right
  InU21 : PMIOPort  Port=21  Side=Right
  OutU21 : PMIOPort  Port=22  Side=Right
  InU31 : PMIOPort  Port=23  Side=Right
  OutU31 : PMIOPort  Port=24  Side=Right
  InD01 : PMIOPort  Port=25  Side=Left
  OutD01 : PMIOPort  Port=26  Side=Left
  InD11 : PMIOPort  Port=27  Side=Left
  OutD11 : PMIOPort  Port=28  Side=Left
  InD21 : PMIOPort  Port=29  Side=Left
  OutD21 : PMIOPort  Port=30  Side=Left
  InD31 : PMIOPort  Port=31  Side=Left
  OutD31 : PMIOPort  Port=32  Side=Left
  InU02 : PMIOPort  Port=33  Side=Right
  OutU02 : PMIOPort  Port=34  Side=Right
  InU12 : PMIOPort  Port=35  Side=Right
  OutU12 : PMIOPort  Port=36  Side=Right
  InU22 : PMIOPort  Port=37  Side=Right
  OutU22 : PMIOPort  Port=38  Side=Right
  InU32 : PMIOPort  Port=39  Side=Right
  OutU32 : PMIOPort  Port=40  Side=Right
  InD02 : PMIOPort  Port=41  Side=Left
  OutD02 : PMIOPort  Port=42  Side=Left
  InD12 : PMIOPort  Port=43  Side=Left
  OutD12 : PMIOPort  Port=44  Side=Left
  InD22 : PMIOPort  Port=45  Side=Left
  OutD22 : PMIOPort  Port=46  Side=Left
  InD32 : PMIOPort  Port=47  Side=Left
  OutD32 : PMIOPort  Port=48  Side=Left
  InU03 : PMIOPort  Port=49  Side=Right
  OutU03 : PMIOPort  Port=50  Side=Right
  InU13 : PMIOPort  Port=51  Side=Right
  OutU13 : PMIOPort  Port=52  Side=Right
  InU23 : PMIOPort  Port=53  Side=Right
  OutU23 : PMIOPort  Port=54  Side=Right
  InU33 : PMIOPort  Port=55  Side=Right
  OutU33 : PMIOPort  Port=56  Side=Right
  InD03 : PMIOPort  Port=57  Side=Left
  OutD03 : PMIOPort  Port=58  Side=Left
  InD13 : PMIOPort  Port=59  Side=Left
  OutD13 : PMIOPort  Port=60  Side=Left
  InD23 : PMIOPort  Port=61  Side=Left
  OutD23 : PMIOPort  Port=62  Side=Left
  InD33 : PMIOPort  Port=63  Side=Left
  OutD33 : PMIOPort  Port=64  Side=Left
  connections:
  Sitch3DXYZ2/RConn4 -- Sitch3DXYZ3/LConn3
  Sitch3DXYZ4/RConn4 -- Sitch3DXYZ5/LConn3
  Sitch3DXYZ12/RConn1 -- Sitch3DXYZ10/LConn2
  Sitch3DXYZ3/LConn2 -- Sitch3DXYZ7/RConn1
  PE30/RConn1 -- Sitch3DXYZ3/LConn7
  Sitch3DXYZ15/RConn3 -- Sitch3DXYZ14/LConn4
  Sitch3DXYZ10/RConn2 -- Sitch3DXYZ12/LConn1
  Sitch3DXYZ1/RConn2 -- Sitch3DXYZ5/LConn1
  Sitch3DXYZ1/RConn4 -- Sitch3DXYZ2/LConn3
  Sitch3DXYZ10/RConn1 -- Sitch3DXYZ6/LConn2
  Sitch3DXYZ7/LConn2 -- Sitch3DXYZ11/RConn1
  Sitch3DXYZ8/RConn1 -- Sitch3DXYZ4/LConn2
  PE20/LConn1 -- Sitch3DXYZ2/RConn7
  Sitch3DXYZ7/RConn3 -- Sitch3DXYZ6/LConn4
  PE21/RConn1 -- Sitch3DXYZ6/LConn7
  PE01/RConn1 -- Sitch3DXYZ4/LConn7
  PE11/RConn1 -- Sitch3DXYZ5/LConn7
  Sitch3DXYZ15/RConn7 -- PE13/LConn1
  Sitch3DXYZ12/LConn7 -- PE23/RConn1
  Sitch3DXYZ12/RConn7 -- PE23/LConn1
  Sitch3DXYZ13/LConn7 -- PE33/RConn1
  Sitch3DXYZ13/RConn7 -- PE33/LConn1
  Sitch3DXYZ9/RConn2 -- Sitch3DXYZ15/LConn1
  Sitch3DXYZ6/RConn3 -- Sitch3DXYZ5/LConn4
  Sitch3DXYZ9/RConn1 -- Sitch3DXYZ5/LConn2
  Sitch3DXYZ7/RConn2 -- Sitch3DXYZ11/LConn1
  Sitch3DXYZ6/RConn2 -- Sitch3DXYZ10/LConn1
  Sitch3DXYZ5/RConn2 -- Sitch3DXYZ9/LConn1
  Sitch3DXYZ10/RConn3 -- Sitch3DXYZ9/LConn4
  Sitch3DXYZ15/RConn1 -- Sitch3DXYZ9/LConn2
  Sitch3DXYZ6/RConn1 -- Sitch3DXYZ2/LConn2
  Sitch3DXYZ11/RConn3 -- Sitch3DXYZ10/LConn4
  Sitch3DXYZ13/RConn1 -- Sitch3DXYZ11/LConn2
  Sitch3DXYZ5/RConn3 -- Sitch3DXYZ4/LConn4
  Sitch3DXYZ2/RConn2 -- Sitch3DXYZ6/LConn1
  Sitch3DXYZ9/RConn3 -- Sitch3DXYZ8/LConn4
  Sitch3DXYZ8/RConn7 -- PE02/LConn1
  Sitch3DXYZ8/LConn7 -- PE02/RConn1
  PE30/LConn1 -- Sitch3DXYZ3/RConn7
  PE31/RConn1 -- Sitch3DXYZ7/LConn7
  PE31/LConn1 -- Sitch3DXYZ7/RConn7
  Sitch3DXYZ6/RConn7 -- PE21/LConn1
  PE11/LConn1 -- Sitch3DXYZ5/RConn7
  PE01/LConn1 -- Sitch3DXYZ4/RConn7
  Sitch3DXYZ1/RConn3 -- Sitch3DXYZ/LConn4
  Sitch3DXYZ11/RConn2 -- Sitch3DXYZ13/LConn1
  PE10/LConn1 -- Sitch3DXYZ1/RConn7
  Sitch3DXYZ8/RConn4 -- Sitch3DXYZ9/LConn3
  Sitch3DXYZ10/RConn4 -- Sitch3DXYZ11/LConn3
  Sitch3DXYZ9/RConn4 -- Sitch3DXYZ10/LConn3
  Sitch3DXYZ14/RConn4 -- Sitch3DXYZ15/LConn3
  Sitch3DXYZ6/RConn4 -- Sitch3DXYZ7/LConn3
  Sitch3DXYZ15/RConn4 -- Sitch3DXYZ12/LConn3
  Sitch3DXYZ12/RConn4 -- Sitch3DXYZ13/LConn3
  Sitch3DXYZ14/RConn1 -- Sitch3DXYZ8/LConn2
  PE10/RConn1 -- Sitch3DXYZ1/LConn7
  Sitch3DXYZ13/RConn3 -- Sitch3DXYZ12/LConn4
  Sitch3DXYZ3/RConn3 -- Sitch3DXYZ2/LConn4
  Sitch3DXYZ3/RConn2 -- Sitch3DXYZ7/LConn1
  Sitch3DXYZ12/RConn3 -- Sitch3DXYZ15/LConn4
  Sitch3DXYZ/RConn7 -- PE00/LConn1
  Sitch3DXYZ/LConn7 -- PE00/RConn1
  Sitch3DXYZ9/RConn7 -- PE12/LConn1
  Sitch3DXYZ9/LConn7 -- PE12/RConn1
  Sitch3DXYZ/RConn2 -- Sitch3DXYZ4/LConn1
  Sitch3DXYZ8/RConn2 -- Sitch3DXYZ14/LConn1
  Sitch3DXYZ2/LConn7 -- PE20/RConn1
  Sitch3DXYZ5/RConn4 -- Sitch3DXYZ6/LConn3
  Sitch3DXYZ/RConn4 -- Sitch3DXYZ1/LConn3
  Sitch3DXYZ4/RConn1 -- Sitch3DXYZ/LConn2
  PE13/RConn1 -- Sitch3DXYZ15/LConn7
  PE03/RConn1 -- Sitch3DXYZ14/LConn7
  PE03/LConn1 -- Sitch3DXYZ14/RConn7
  Sitch3DXYZ5/RConn1 -- Sitch3DXYZ1/LConn2
  Sitch3DXYZ4/RConn2 -- Sitch3DXYZ8/LConn1
  Sitch3DXYZ2/RConn3 -- Sitch3DXYZ1/LConn4
  PE32/LConn1 -- Sitch3DXYZ11/RConn7
  PE32/RConn1 -- Sitch3DXYZ11/LConn7
  PE22/LConn1 -- Sitch3DXYZ10/RConn7
  PE22/RConn1 -- Sitch3DXYZ10/LConn7
  Sitch3DXYZ15/LConn6 -- InD13/RConn1
  Sitch3DXYZ/RConn5 -- OutU00/RConn1
  Sitch3DXYZ15/RConn6 -- OutD13/RConn1
  Sitch3DXYZ2/LConn5 -- InU20/RConn1
  Sitch3DXYZ8/LConn5 -- InU02/RConn1
  Sitch3DXYZ11/LConn6 -- InD32/RConn1
  Sitch3DXYZ15/RConn5 -- OutU13/RConn1
  Sitch3DXYZ7/RConn5 -- OutU31/RConn1
  Sitch3DXYZ12/RConn5 -- OutU23/RConn1
  Sitch3DXYZ15/LConn5 -- InU13/RConn1
  Sitch3DXYZ14/LConn6 -- InD03/RConn1
  Sitch3DXYZ3/RConn5 -- OutU30/RConn1
  Sitch3DXYZ14/RConn5 -- OutU03/RConn1
  Sitch3DXYZ/LConn6 -- InD00/RConn1
  Sitch3DXYZ13/LConn5 -- InU33/RConn1
  Sitch3DXYZ14/LConn5 -- InU03/RConn1
  Sitch3DXYZ11/RConn5 -- OutU32/RConn1
  Sitch3DXYZ11/LConn5 -- InU32/RConn1
  Sitch3DXYZ5/RConn6 -- OutD11/RConn1
  Sitch3DXYZ11/RConn6 -- OutD32/RConn1
  Sitch3DXYZ3/LConn6 -- InD30/RConn1
  Sitch3DXYZ8/LConn6 -- InD02/RConn1
  Sitch3DXYZ12/LConn6 -- InD23/RConn1
  Sitch3DXYZ3/LConn5 -- InU30/RConn1
  Sitch3DXYZ8/RConn5 -- OutU02/RConn1
  Sitch3DXYZ7/LConn6 -- InD31/RConn1
  Sitch3DXYZ8/RConn6 -- OutD02/RConn1
  Sitch3DXYZ13/RConn6 -- OutD33/RConn1
  Sitch3DXYZ2/RConn6 -- OutD20/RConn1
  Sitch3DXYZ5/RConn5 -- OutU11/RConn1
  Sitch3DXYZ12/RConn6 -- OutD23/RConn1
  Sitch3DXYZ3/RConn6 -- OutD30/RConn1
  Sitch3DXYZ13/RConn5 -- OutU33/RConn1
  Sitch3DXYZ2/RConn5 -- OutU20/RConn1
  Sitch3DXYZ12/LConn5 -- InU23/RConn1
  Sitch3DXYZ/LConn5 -- InU00/RConn1
  Sitch3DXYZ5/LConn5 -- InU11/RConn1
  Sitch3DXYZ7/LConn5 -- InU31/RConn1
  Sitch3DXYZ7/RConn6 -- OutD31/RConn1
  Sitch3DXYZ5/LConn6 -- InD11/RConn1
  Sitch3DXYZ13/LConn6 -- InD33/RConn1
  Sitch3DXYZ2/LConn6 -- InD20/RConn1
  Sitch3DXYZ/RConn6 -- OutD00/RConn1
  Sitch3DXYZ14/RConn6 -- OutD03/RConn1
  Sitch3DXYZ6/LConn5 -- InU21/RConn1
  Sitch3DXYZ6/LConn6 -- InD21/RConn1
  Sitch3DXYZ6/RConn5 -- OutU21/RConn1
  Sitch3DXYZ6/RConn6 -- OutD21/RConn1
  Sitch3DXYZ10/LConn5 -- InU22/RConn1
  Sitch3DXYZ10/LConn6 -- InD22/RConn1
  Sitch3DXYZ10/RConn5 -- OutU22/RConn1
  Sitch3DXYZ10/RConn6 -- OutD22/RConn1
  Sitch3DXYZ1/LConn5 -- InU10/RConn1
  Sitch3DXYZ1/LConn6 -- InD10/RConn1
  Sitch3DXYZ1/RConn5 -- OutU10/RConn1
  Sitch3DXYZ1/RConn6 -- OutD10/RConn1
  Sitch3DXYZ4/LConn5 -- InU01/RConn1
  Sitch3DXYZ4/LConn6 -- InD01/RConn1
  Sitch3DXYZ4/RConn5 -- OutU01/RConn1
  Sitch3DXYZ4/RConn6 -- OutD01/RConn1
  Sitch3DXYZ9/LConn5 -- InU12/RConn1
  Sitch3DXYZ9/LConn6 -- InD12/RConn1
  Sitch3DXYZ9/RConn5 -- OutU12/RConn1
  Sitch3DXYZ9/RConn6 -- OutD12/RConn1
